simulink model "NewFullAM_Mod_Dem"  (R2023a)
settings: Solver=ode45  StartTime=0.0  StopTime=1  RelTol=1e-3
libraries: dspfdesign x1
settings Model: Creator=Pedro  LastModifiedBy=Pedro

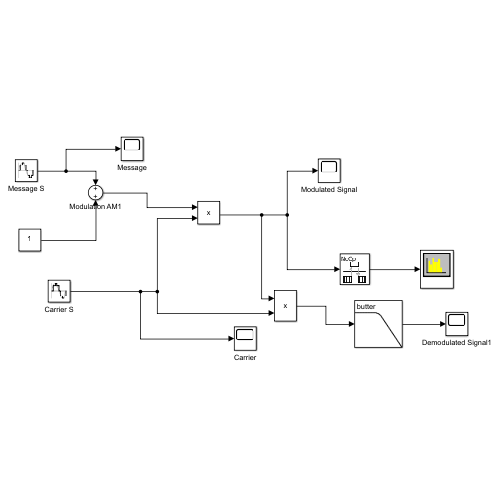
[thumbnail: Simulink's stored preview of the top-level diagram]
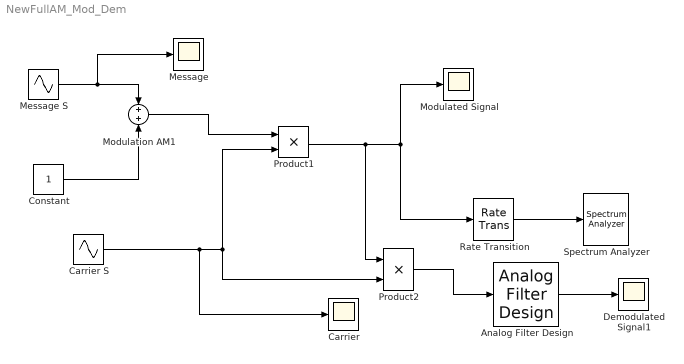
== system NewFullAM_Mod_Dem ==
  Analog Filter Design : dspfdesign/Analog Filter Design  method=Butterworth  filttype=Lowpass  N=4  Wlo=30  Whi=80  Rp=2  Rs=40
  Carrier : Scope
  Carrier S : Sin  Amplitude=3  Frequency=2*pi*27  SampleTime=1/1000
  Constant : Constant
  Demodulated Signal1 : Scope
  Message : Scope
  Message S : Sin  Frequency=2*pi*2  SampleTime=1/1000
  Modulated Signal : Scope
  Modulation AM1 : Sum
  Product1 : Product
  Product2 : Product
  Rate Transition : RateTransition  OutPortSampleTime=0.001
  Spectrum Analyzer : SpectrumAnalyzer  WindowPosition=[1.000000,41.000000,1280.000000,657.000000,]  ScopeFrameLocation=window  SampleRateSource=Property  SampleRate=44.1e3  PlotAsTwoSidedSpectrum=off  FrequencyScale=Log  FrequencySpan=Start and stop frequencies  StartFrequency=20  StopFrequency=20e3  SpectrumUnits=Watts  YLimits=[-224.69097444,6.5417711]  ColorLimits=[-20 80]  SelectedToolstripTab=spectrumAnalyzerToolstrip.spectrumTab  DefaultConfigurationName=spbscopes.SpectrumAnalyzerBlockCfg  IsFrequencyInputMode=0  FrequencyVectorPort=0  FrequencyVectorFromPort=0  FrequencyInputRBWPort=0  FrequencyInputRBWFromPort=0
  wires:
  Carrier S/1 -> Carrier/1, Product2/2, Product1/2
  Constant/1 -> Modulation AM1/2
  Modulation AM1/1 -> Product1/1
  Product1/1 -> Product2/1, Rate Transition/1, Modulated Signal/1
  Message S/1 -> Message/1, Modulation AM1/1
  Product2/1 -> Analog Filter Design/1
  Analog Filter Design/1 -> Demodulated Signal1/1
  Rate Transition/1 -> Spectrum Analyzer/1
